simulink model "sampleModel20"  (R2021a)
settings: Solver=VariableStepAuto  StartTime=0.0  StopTime=10.0  RelTol=1e-3
undefined symbols (not defined in the file): DiscIntNeverNeededParam, magnitude, Newton, Raphson
libraries: simulink x274, pid_lib x17
(part 9 of 16)

== system sampleModel20/cfblk77/cfblk5/cfblk9/cfblk9 ==
  cfblk1 : Inport
  cfblk10 : Inport  Port=2
  cfblk3 : Math  Operator=mod  SaturateOnIntegerOverflow=on
  cfblk4 : Sum  Inputs=|++
  cfblk5 : Bias  Bias=[-186657263.890599]
  cfblk6 : Abs
  cfblk7 : Bias  Bias=[-144051976.581815]
  cfblk8 : Sum  Inputs=|++
  cfblk9 : simulink/Math Operations/MinMax Running Resettable  Function=min  vinit=0.0
  cfblk2 : Outport
  wires:
  cfblk10/1 -> cfblk6/1
  cfblk8/1 -> cfblk3/1
  cfblk9/1 -> cfblk5/1
  cfblk1/1 -> cfblk8/1
  cfblk5/1 -> cfblk2/1
  cfblk4/1 -> cfblk8/2
  cfblk6/1 -> cfblk7/1, cfblk4/2, cfblk3/2
  cfblk7/1 -> cfblk9/1, cfblk4/1
  cfblk3/1 -> cfblk9/2

== system sampleModel20/cfblk77/cfblk6/cfblk5/cfblk9 ==
  cfblk1 : Inport
  cfblk7 : Inport  Port=2
  cfblk8 : Inport  Port=3
  cfblk9 : Inport  Port=4
  cfblk13 : Delay  SampleTime=1
  cfblk14 : Delay  SampleTime=1
  cfblk3 : DiscreteTransferFcn  SampleTime=1
  cfblk4 : ComplexToRealImag
  cfblk5 : Gain  Gain=[186657996.322162]
  cfblk6 : Sum  Inputs=+
  cfblk2 : Outport
  cfblk10 : Outport  Port=2
  cfblk11 : Outport  Port=3
  cfblk12 : Outport  Port=4
  wires:
  cfblk3/1 -> cfblk5/1
  cfblk7/1 -> cfblk2/1
  cfblk8/1 -> cfblk11/1
  cfblk4/1 -> cfblk6/1
  cfblk9/1 -> cfblk10/1
  cfblk4/2 -> cfblk12/1
  cfblk5/1 -> cfblk13/1
  cfblk13/1 -> cfblk3/1
  cfblk6/1 -> cfblk14/1
  cfblk14/1 -> cfblk4/1

== system sampleModel20/cfblk77/cfblk6/cfblk6/cfblk6 ==
  cfblk1 : Inport
  cfblk4 : Inport  Port=2
  cfblk5 : Inport  Port=3
  cfblk6 : Inport  Port=4
  cfblk3 : Sin  TimeSource=Use external signal  SampleTime=0
  cfblk2 : Outport
  cfblk7 : Outport  Port=2
  wires:
  cfblk5/1 -> cfblk3/1
  cfblk1/1 -> cfblk2/1
  cfblk6/1 -> cfblk7/1

== system sampleModel20/cfblk77/cfblk6/cfblk6/cfblk7 ==
  cfblk1 : Inport
  cfblk10 : Inport  Port=2
  cfblk11 : Inport  Port=3
  cfblk12 : Inport  Port=4
  cfblk13 : Inport  Port=5
  cfblk14 : Inport  Port=6
  cfblk3 : ComplexToRealImag
  cfblk4 : Sqrt  Operator=rSqrt  AlgorithmType=Newton-Raphson  SaturateOnIntegerOverflow=on
  cfblk5 : PermuteDimensions
  cfblk6 : Reshape
  cfblk7 : Sum  Inputs=+
  cfblk8 : Product  Inputs=*
  cfblk9 : Sum  Inputs=|++
  cfblk2 : Outport
  cfblk15 : Outport  Port=2
  wires:
  cfblk13/1 -> cfblk15/1
  cfblk3/1 -> cfblk4/1
  cfblk10/1 -> cfblk8/1
  cfblk1/1 -> cfblk7/1
  cfblk9/1 -> cfblk5/1
  cfblk3/2 -> cfblk9/1
  cfblk5/1 -> cfblk6/1
  cfblk7/1 -> cfblk2/1
  cfblk12/1 -> cfblk3/1
  cfblk4/1 -> cfblk9/2

== system sampleModel20/cfblk77/cfblk6/cfblk6/cfblk8 ==
  cfblk1 : Inport
  cfblk12 : Inport  Port=2
  cfblk13 : Inport  Port=3
  cfblk14 : Inport  Port=4
  cfblk15 : Inport  Port=5
  cfblk16 : Inport  Port=6
  cfblk10 : Sum  Inputs=+-
  cfblk11 : Gain  Gain=[-598651231.399179]
  cfblk18 : Delay  SampleTime=1
  cfblk3 : Product  Inputs=**
  cfblk4 : Product  Inputs=**
  cfblk5 : Assignment  DiagnosticForDimensions=Warning  IndexOptions=Index vector (dialog)  Indices=1  OutputSizes=1
  cfblk6 : Assignment  DiagnosticForDimensions=Warning  IndexOptions=Index vector (dialog)  Indices=1  OutputSizes=1
  cfblk7 : Abs
  cfblk8 : Bias  Bias=[-168883268.146316]
  cfblk9 : Sum  Inputs=|++
  cfblk2 : Outport
  cfblk17 : Outport  Port=2
  wires:
  cfblk15/1 -> cfblk9/1
  cfblk14/1 -> cfblk3/1
  cfblk16/1 -> cfblk6/1, cfblk10/2
  cfblk5/1 -> cfblk11/1
  cfblk13/1 -> cfblk17/1
  cfblk4/1 -> cfblk6/2
  cfblk12/1 -> cfblk5/1
  cfblk11/1 -> cfblk2/1
  cfblk1/1 -> cfblk9/2
  cfblk10/1 -> cfblk4/2
  cfblk6/1 -> cfblk8/1
  cfblk9/1 -> cfblk7/1
  cfblk3/1 -> cfblk10/1
  cfblk7/1 -> cfblk3/2, cfblk5/2
  cfblk8/1 -> cfblk18/1
  cfblk18/1 -> cfblk4/1

== system sampleModel20/cfblk77/cfblk6/cfblk7/cfblk11 ==
  cfblk1 : Inport
  cfblk8 : Inport  Port=2
  cfblk9 : Inport  Port=3
  cfblk10 : Inport  Port=4
  cfblk11 : Inport  Port=5
  cfblk12 : Inport  Port=6
  cfblk3 : simulink/Math Operations/Slider Gain  gain=1  low=0  high=2
  cfblk4 : Sum  Inputs=|++
  cfblk5 : Sqrt  SaturateOnIntegerOverflow=on
  cfblk6 : ComplexToRealImag
  cfblk7 : Rounding
  cfblk2 : Outport
  cfblk13 : Outport  Port=2
  wires:
  cfblk6/1 -> cfblk7/1
  cfblk5/1 -> cfblk6/1
  cfblk8/1 -> cfblk2/1
  cfblk12/1 -> cfblk5/1
  cfblk10/1 -> cfblk4/1
  cfblk1/1 -> cfblk4/2
  cfblk11/1 -> cfblk3/1
  cfblk9/1 -> cfblk13/1

== system sampleModel20/cfblk77/cfblk6/cfblk7/cfblk12 ==
  cfblk1 : Inport
  cfblk7 : Inport  Port=2
  cfblk8 : Inport  Port=3
  cfblk3 : Reshape
  cfblk4 : Sum  Inputs=|++
  cfblk5 : Rounding
  cfblk6 : Sqrt  Operator=rSqrt  AlgorithmType=Newton-Raphson  SaturateOnIntegerOverflow=on
  cfblk9 : Delay  SampleTime=1
  cfblk2 : Outport
  wires:
  cfblk8/1 -> cfblk2/1
  cfblk5/1 -> cfblk4/1
  cfblk1/1 -> cfblk5/1
  cfblk7/1 -> cfblk3/1
  cfblk4/1 -> cfblk6/1
  cfblk6/1 -> cfblk9/1
  cfblk9/1 -> cfblk4/2

== system sampleModel20/cfblk77/cfblk6/cfblk8/cfblk8 ==
  cfblk1 : Inport
  cfblk5 : Inport  Port=2
  cfblk6 : Inport  Port=3
  cfblk7 : Inport  Port=4
  cfblk8 : Inport  Port=5
  cfblk9 : Inport  Port=6
  cfblk10 : Inport  Port=7
  cfblk3 : Product  Inputs=*
  cfblk4 : simulink/Math Operations/MinMax Running Resettable  Function=min  vinit=0.0
  cfblk2 : Outport
  cfblk11 : Outport  Port=2
  wires:
  cfblk4/1 -> cfblk3/1
  cfblk5/1 -> cfblk2/1
  cfblk10/1 -> cfblk4/1
  cfblk9/1 -> cfblk11/1
  cfblk1/1 -> cfblk4/2

== system sampleModel20/cfblk77/cfblk6/cfblk8/cfblk9 ==
  cfblk1 : Inport
  cfblk4 : Inport  Port=2
  cfblk5 : Inport  Port=3
  cfblk6 : Inport  Port=4
  cfblk3 : Bias  Bias=[-292302917.614101]
  cfblk2 : Outport
  cfblk7 : Outport  Port=2
  wires:
  cfblk4/1 -> cfblk2/1
  cfblk6/1 -> cfblk7/1
  cfblk5/1 -> cfblk3/1

== system sampleModel20/cfblk77/cfblk6/cfblk9/cfblk7 ==
  cfblk1 : Inport
  cfblk6 : Inport  Port=2
  cfblk7 : Inport  Port=3
  cfblk8 : Inport  Port=4
  cfblk9 : Inport  Port=5
  cfblk10 : Inport  Port=6
  cfblk11 : Inport  Port=7
  cfblk3 : MinMax  Function=max  Inputs=3
  cfblk4 : Product
  cfblk5 : Trigonometry
  cfblk2 : Outport
  cfblk12 : Outport  Port=2
  cfblk13 : Outport  Port=3
  cfblk14 : Outport  Port=4
  wires:
  cfblk1/1 -> cfblk5/1
  cfblk4/1 -> cfblk12/1
  cfblk5/1 -> cfblk4/1
  cfblk6/1 -> cfblk4/2
  cfblk10/1 -> cfblk3/1
  cfblk3/1 -> cfblk13/1
  cfblk7/1 -> cfblk2/1
  cfblk11/1 -> cfblk14/1
  cfblk9/1 -> cfblk3/2
  cfblk8/1 -> cfblk3/3

== system sampleModel20/cfblk77/cfblk6/cfblk9/cfblk8 ==
  cfblk1 : Inport
  cfblk5 : Inport  Port=2
  cfblk6 : Inport  Port=3
  cfblk3 : Squeeze
  cfblk4 : ComplexToMagnitudeAngle
  cfblk2 : Outport
  cfblk7 : Outport  Port=2
  wires:
  cfblk1/1 -> cfblk7/1
  cfblk4/1 -> cfblk2/1
  cfblk5/1 -> cfblk3/1
  cfblk3/1 -> cfblk4/1

== system sampleModel20/cfblk77/cfblk7/cfblk10/cfblk10 ==
  cfblk1 : Inport
  cfblk6 : Inport  Port=2
  cfblk7 : Inport  Port=3
  cfblk8 : Inport  Port=4
  cfblk9 : Inport  Port=5
  cfblk3 : simulink/Math Operations/MinMax Running Resettable  Function=min  vinit=0.0
  cfblk4 : ComplexToMagnitudeAngle
  cfblk5 : Gain  Gain=[652238342.291025]
  cfblk2 : Outport
  wires:
  cfblk4/1 -> cfblk5/1
  cfblk9/1 -> cfblk4/1
  cfblk4/2 -> cfblk2/1
  cfblk5/1 -> cfblk3/1
  cfblk7/1 -> cfblk3/2

== system sampleModel20/cfblk77/cfblk7/cfblk10/cfblk11 ==
  cfblk1 : Inport
  cfblk5 : Inport  Port=2
  cfblk6 : Inport  Port=3
  cfblk3 : Delay  ShowEnablePort=on  SampleTime=1
      settings: InputPortMap=u0,e6
  cfblk4 : UnaryMinus
  cfblk8 : Delay  SampleTime=1
  cfblk2 : Outport
  cfblk7 : Outport  Port=2
  wires:
  cfblk3/1 -> cfblk4/1
  cfblk5/1 -> cfblk7/1
  cfblk1/1 -> cfblk2/1
  cfblk6/1 -> cfblk3/1
  cfblk4/1 -> cfblk8/1
  cfblk8/1 -> cfblk3/2

== system sampleModel20/cfblk77/cfblk7/cfblk10/cfblk12 ==
  cfblk1 : Inport
  cfblk12 : Inport  Port=2
  cfblk13 : Inport  Port=3
  cfblk14 : Inport  Port=4
  cfblk10 : Polyval  Coefs=[ +2.081618890e-019, -1.441693666e-014, +4.719686976e-010, -8.536869453e-006, +1.621573104e-001, -8.087801117e+001 ]
  cfblk11 : Abs
  cfblk3 : pid_lib/PID Controller  Controller=PID  Form=Parallel  TimeDomain=Discrete-time  UseExternalTs=off  SampleTime=1  IntegratorMethod=Forward Euler  FilterMethod=Forward Euler  ControllerParametersSource=internal  P=1  I=1  D=0  UseFilter=on  N=100  TunerSelectOption=Transfer Function Based (PID Tuner App)  InitialConditionSource=internal  InitialConditionForIntegrator=0  InitialConditionForFilter=0  DifferentiatorICPrevScaledInput=0  ExternalReset=none  TrackingMode=off  Kt=1  LimitOutput=off  SatLimitsSource=internal  UpperSaturationLimit=inf  LowerSaturationLimit=-inf  LinearizeAsGain=off  AntiWindupMode=none  Kb=1  POutMin=[]  POutMax=[]  IOutMin=[]  IOutMax=[]  DOutMin=[]  DOutMax=[]  NOutMin=[]  NOutMax=[]  SumOutMin=[]  SumOutMax=[]  SaturationOutMin=[]  SaturationOutMax=[]  PParamMin=[]  PParamMax=[]  IParamMin=[]  IParamMax=[]  DParamMin=[]  DParamMax=[]  NParamMin=[]  NParamMax=[]  KbParamMin=[]  KbParamMax=[]  KtParamMin=[]  KtParamMax=[]  KbOutMin=[]  KbOutMax=[]  KtOutMin=[]  KtOutMax=[]  IntegratorOutMin=[]  IntegratorOutMax=[]  FilterOutMin=[]  FilterOutMax=[]  SumI1OutMin=[]  SumI1OutMax=[]  SumI2OutMin=[]  SumI2OutMax=[]  SumI3OutMin=[]  SumI3OutMax=[]  SumI4OutMin=[]  SumI4OutMax=[]  SumDOutMin=[]  SumDOutMax=[]  DifferentiatorOutMin=[]  DifferentiatorOutMax=[]  FilterDiffOutCoefMin=[]  FilterDiffOutCoefMax=[]  ReciprocalOutMin=[]  ReciprocalOutMax=[]  SumDenOutMin=[]  SumDenOutMax=[]  SumNumOutMin=[]  SumNumOutMax=[]  DivideOutMin=[]  DivideOutMax=[]  UdiffTsProdOutMin=[]  UdiffTsProdOutMax=[]  NTsProdOutMin=[]  NTsProdOutMax=[]  UintegralTsProdOutMin=[]  UintegralTsProdOutMax=[]  UngainTsProdOutMin=[]  UngainTsProdOutMax=[]  IntegratorContinuousStateAttributes=''  IntegratorStateMustResolveToSignalObject=off  IntegratorRTWStateStorageClass=Auto  FilterContinuousStateAttributes=''  FilterStateMustResolveToSignalObject=off  FilterRTWStateStorageClass=Auto  ParallelPVariant=InternalParameters  IdealPVariant=Disabled  IVariant=InternalParameters  DVariant=InternalParameters  IntegratorVariant=Discrete  SatVariant=Disabled  AWVariant=Passthrough  PCopyVariant=Disabled  TRVariant=Disabled  FdbkBlocksVariant=Forward  IdealPFdbkVariant=Disabled  SatFdbkVariant=Disabled  DerivativeFilterVariant=ForwardEulerFilter  NVariant=InternalParameters  NCopyVariant=Disabled  FilterICVariant=InternalICsFilter  IntegratorICVariant=InternalICs  ExternalResetVariant=Disabled  TRSumVariant=Passthrough  SumFdbkVariant=Disabled  SumVariant=Sum_PID  TsampFilterVariant=InternalTs  TsampNgainVariant=Passthrough  TsampIntegralVariant=Passthrough  ExternalSaturationOutDataTypeStr=Inherit: Same as second input
  cfblk4 : Product  Inputs=*
  cfblk5 : Squeeze
  cfblk6 : PermuteDimensions
  cfblk7 : Squeeze
  cfblk8 : Product  Inputs=*
  cfblk9 : ComplexToMagnitudeAngle
  cfblk2 : Outport
  cfblk15 : Outport  Port=2
  cfblk16 : Outport  Port=3
  cfblk17 : Outport  Port=4
  wires:
  cfblk3/1 -> cfblk9/1
  cfblk4/1 -> cfblk8/1
  cfblk5/1 -> cfblk11/1
  cfblk11/1 -> cfblk3/1
  cfblk1/1 -> cfblk6/1
  cfblk14/1 -> cfblk15/1
  cfblk8/1 -> cfblk7/1
  cfblk7/1 -> cfblk16/1
  cfblk6/1 -> cfblk2/1
  cfblk12/1 -> cfblk5/1
  cfblk13/1 -> cfblk10/1
  cfblk9/1 -> cfblk17/1
  cfblk9/2 -> cfblk4/1

== system sampleModel20/cfblk77/cfblk7/cfblk10/cfblk13 ==
  cfblk1 : Inport
  cfblk9 : Inport  Port=2
  cfblk10 : Inport  Port=3
  cfblk11 : Inport  Port=4
  cfblk12 : Inport  Port=5
  cfblk13 : Inport  Port=6
  cfblk14 : Inport  Port=7
  cfblk3 : simulink/Discrete/Difference  ICPrevInput=0.0  OutMin=[]  OutMax=[]  OutDataTypeStr=Inherit: Inherit via back propagation  OutDataType=fixdt(1, 16)  OutScaling=2^-10  DoSatur=off
  cfblk4 : Sqrt  Operator=rSqrt  AlgorithmType=Newton-Raphson  SaturateOnIntegerOverflow=on
  cfblk5 : Sum  Inputs=|++
  cfblk6 : Trigonometry
  cfblk7 : ComplexToMagnitudeAngle
  cfblk8 : UnaryMinus
  cfblk2 : Outport
  cfblk15 : Outport  Port=2
  cfblk16 : Outport  Port=3
  cfblk17 : Outport  Port=4
  wires:
  cfblk13/1 -> cfblk17/1
  cfblk1/1 -> cfblk8/1
  cfblk10/1 -> cfblk5/1
  cfblk8/1 -> cfblk3/1
  cfblk12/1 -> cfblk15/1
  cfblk9/1 -> cfblk4/1
  cfblk11/1 -> cfblk16/1
  cfblk14/1 -> cfblk7/1
  cfblk4/1 -> cfblk6/1
  cfblk7/1 -> cfblk5/2
  cfblk6/1 -> cfblk2/1

== system sampleModel20/cfblk77/cfblk7/cfblk10/cfblk9 ==
  cfblk1 : Inport
  cfblk8 : Inport  Port=2
  cfblk9 : Inport  Port=3
  cfblk10 : Inport  Port=4
  cfblk11 : Inport  Port=5
  cfblk12 : Inport  Port=6
  cfblk13 : Inport  Port=7
  cfblk14 : Delay  SampleTime=1
  cfblk3 : Reshape
  cfblk4 : Sin  TimeSource=Use external signal  SampleTime=0
  cfblk5 : Abs
  cfblk6 : Bias  Bias=[-31221541.110679]
  cfblk7 : Product
  cfblk2 : Outport
  wires:
  cfblk1/1 -> cfblk2/1
  cfblk11/1 -> cfblk6/1
  cfblk13/1 -> cfblk7/1
  cfblk12/1 -> cfblk4/1
  cfblk3/1 -> cfblk7/2
  cfblk10/1 -> cfblk5/1
  cfblk7/1 -> cfblk14/1
  cfblk14/1 -> cfblk3/1

== system sampleModel20/cfblk77/cfblk7/cfblk8/cfblk7 ==
  cfblk1 : Inport
  cfblk7 : Inport  Port=2
  cfblk8 : Inport  Port=3
  cfblk9 : Inport  Port=4
  cfblk10 : Inport  Port=5
  cfblk11 : Inport  Port=6
  cfblk12 : Inport  Port=7
  cfblk13 : Inport  Port=8
  cfblk3 : DiscreteFir  SampleTime=1
  cfblk4 : Gain  Gain=[-495455232.000155]
  cfblk5 : Squeeze
  cfblk6 : ComplexToMagnitudeAngle
  cfblk2 : Outport
  cfblk14 : Outport  Port=2
  wires:
  cfblk11/1 -> cfblk5/1
  cfblk8/1 -> cfblk6/1
  cfblk1/1 -> cfblk3/1
  cfblk9/1 -> cfblk4/1
  cfblk5/1 -> cfblk2/1
  cfblk7/1 -> cfblk14/1

== system sampleModel20/cfblk77/cfblk7/cfblk8/cfblk8 ==
  cfblk1 : Inport
  cfblk5 : Inport  Port=2
  cfblk6 : Inport  Port=3
  cfblk7 : Inport  Port=4
  cfblk8 : Inport  Port=5
  cfblk3 : Math  Operator=mod  SaturateOnIntegerOverflow=on
  cfblk4 : Rounding
  cfblk2 : Outport
  cfblk9 : Outport  Port=2
  wires:
  cfblk4/1 -> cfblk3/1
  cfblk7/1 -> cfblk3/2
  cfblk1/1 -> cfblk9/1
  cfblk8/1 -> cfblk4/1
  cfblk6/1 -> cfblk2/1

== system sampleModel20/cfblk77/cfblk7/cfblk8/cfblk9 ==
  cfblk1 : Inport
  cfblk7 : Inport  Port=2
  cfblk8 : Inport  Port=3
  cfblk3 : simulink/Math Operations/Slider Gain  gain=1  low=0  high=2
  cfblk4 : Polyval  Coefs=[ +2.081618890e-019, -1.441693666e-014, +4.719686976e-010, -8.536869453e-006, +1.621573104e-001, -8.087801117e+001 ]
  cfblk5 : DotProduct  InputSameDT=on  OutDataTypeStr=Inherit: Inherit via internal rule
  cfblk6 : ComplexToRealImag
  cfblk2 : Outport
  cfblk9 : Outport  Port=2
  wires:
  cfblk7/1 -> cfblk3/1
  cfblk1/1 -> cfblk6/1
  cfblk6/1 -> cfblk2/1
  cfblk6/2 -> cfblk4/1
  cfblk3/1 -> cfblk5/1
  cfblk8/1 -> cfblk9/1
  cfblk4/1 -> cfblk5/2

== system sampleModel20/cfblk77/cfblk7/cfblk9/cfblk18 ==
  cfblk1 : Inport
  cfblk6 : Inport  Port=2
  cfblk7 : Inport  Port=3
  Action Port : ActionPort  ActionPortLabel=if(u1 >= 0)
  cfblk3 : ComplexToMagnitudeAngle
  cfblk4 : PermuteDimensions
  cfblk5 : Polyval  Coefs=[ +2.081618890e-019, -1.441693666e-014, +4.719686976e-010, -8.536869453e-006, +1.621573104e-001, -8.087801117e+001 ]
  cfblk2 : Outport
  wires:
  cfblk6/1 -> cfblk5/1
  cfblk5/1 -> cfblk4/1
  cfblk3/1 -> cfblk2/1
  cfblk7/1 -> cfblk3/1

== system sampleModel20/cfblk77/cfblk7/cfblk9/cfblk19 ==
  cfblk1 : Inport
  cfblk6 : Inport  Port=2
  cfblk7 : Inport  Port=3
  Action Port : ActionPort  ActionPortLabel=else
  cfblk3 : Product  Inputs=*
  cfblk4 : Sin  TimeSource=Use external signal  SampleTime=0
  cfblk5 : MinMax  Inputs=3
  cfblk2 : Outport
  wires:
  cfblk1/1 -> cfblk3/1
  cfblk6/1 -> cfblk4/1
  cfblk3/1 -> cfblk2/1
  cfblk4/1 -> cfblk5/1
  cfblk7/1 -> cfblk5/2, cfblk5/3

== system sampleModel20/cfblk77/cfblk7/cfblk9/cfblk8 ==
  cfblk1 : Inport
  cfblk10 : Inport  Port=2
  cfblk11 : Inport  Port=3
  cfblk12 : Inport  Port=4
  cfblk13 : Inport  Port=5
  cfblk14 : Inport  Port=6
  cfblk3 : Trigonometry
  cfblk4 : Polyval  Coefs=[ +2.081618890e-019, -1.441693666e-014, +4.719686976e-010, -8.536869453e-006, +1.621573104e-001, -8.087801117e+001 ]
  cfblk5 : Assignment  DiagnosticForDimensions=Warning  IndexOptions=Index vector (dialog)  Indices=1  OutputSizes=1
  cfblk6 : Trigonometry
  cfblk7 : Product
  cfblk8 : Signum
  cfblk9 : Reshape
  cfblk2 : Outport
  cfblk15 : Outport  Port=2
  wires:
  cfblk4/1 -> cfblk6/1
  cfblk5/1 -> cfblk15/1
  cfblk6/1 -> cfblk7/1
  cfblk14/1 -> cfblk4/1
  cfblk11/1 -> cfblk3/1
  cfblk1/1 -> cfblk9/1
  cfblk8/1 -> cfblk2/1
  cfblk3/1 -> cfblk7/2
  cfblk9/1 -> cfblk8/1
  cfblk10/1 -> cfblk5/1
  cfblk7/1 -> cfblk5/2

== system sampleModel20/cfblk77/cfblk7/cfblk9/cfblk9 ==
  cfblk1 : Inport
  cfblk11 : Inport  Port=2
  cfblk12 : Inport  Port=3
  cfblk13 : Inport  Port=4
  cfblk14 : Inport  Port=5
  cfblk10 : simulink/Math Operations/MinMax Running Resettable  Function=min  vinit=0.0
  cfblk3 : Reshape
  cfblk4 : Squeeze
  cfblk5 : Sqrt  SaturateOnIntegerOverflow=on
  cfblk6 : Sum  Inputs=+
  cfblk7 : Assignment  DiagnosticForDimensions=Warning  IndexOptions=Index vector (dialog)  Indices=1  OutputSizes=1
  cfblk8 : Abs
  cfblk9 : simulink/Math Operations/MinMax Running Resettable  Function=min  vinit=0.0
  cfblk2 : Outport
  cfblk15 : Outport  Port=2
  cfblk16 : Outport  Port=3
  cfblk17 : Outport  Port=4
  wires:
  cfblk3/1 -> cfblk16/1
  cfblk11/1 -> cfblk9/1
  cfblk12/1 -> cfblk7/1
  cfblk8/1 -> cfblk2/1
  cfblk1/1 -> cfblk4/1
  cfblk13/1 -> cfblk5/1
  cfblk7/1 -> cfblk8/1
  cfblk5/1 -> cfblk10/1
  cfblk4/1 -> cfblk9/2, cfblk7/2
  cfblk14/1 -> cfblk15/1
  cfblk6/1 -> cfblk17/1
  cfblk9/1 -> cfblk10/2
  cfblk10/1 -> cfblk6/1, cfblk3/1

== system sampleModel20/cfblk77/cfblk8/cfblk10/cfblk7 ==
  cfblk1 : Inport
  cfblk6 : Inport  Port=2
  cfblk7 : Inport  Port=3
  cfblk8 : Inport  Port=4
  cfblk9 : Inport  Port=5
  cfblk10 : Inport  Port=6
  cfblk11 : Inport  Port=7
  cfblk12 : Inport  Port=8
  cfblk15 : Delay  SampleTime=1
  cfblk3 : Sum  Inputs=+-
  cfblk4 : Product  Inputs=*
  cfblk5 : DotProduct  InputSameDT=on  OutDataTypeStr=Inherit: Inherit via internal rule
  cfblk2 : Outport
  cfblk13 : Outport  Port=2
  cfblk14 : Outport  Port=3
  wires:
  cfblk5/1 -> cfblk4/1
  cfblk6/1 -> cfblk14/1
  cfblk12/1 -> cfblk3/1
  cfblk7/1 -> cfblk13/1
  cfblk1/1 -> cfblk5/1
  cfblk8/1 -> cfblk2/1
  cfblk11/1 -> cfblk3/2
  cfblk4/1 -> cfblk15/1
  cfblk15/1 -> cfblk5/2

== system sampleModel20/cfblk77/cfblk8/cfblk10/cfblk8 ==
  cfblk1 : Inport
  cfblk9 : Inport  Port=2
  cfblk10 : Inport  Port=3
  cfblk11 : Inport  Port=4
  cfblk14 : Delay  SampleTime=1
  cfblk15 : Delay  SampleTime=1
  cfblk3 : Product
  cfblk4 : ComplexToMagnitudeAngle
  cfblk5 : Squeeze
  cfblk6 : ComplexToMagnitudeAngle
  cfblk7 : simulink/Math Operations/Slider Gain  gain=1  low=0  high=2
  cfblk8 : ComplexToMagnitudeAngle
  cfblk2 : Outport
  cfblk12 : Outport  Port=2
  cfblk13 : Outport  Port=3
  wires:
  cfblk5/1 -> cfblk2/1
  cfblk3/1 -> cfblk8/1
  cfblk6/1 -> cfblk3/2
  cfblk6/2 -> cfblk7/1
  cfblk11/1 -> cfblk5/1
  cfblk4/1 -> cfblk13/1
  cfblk1/1 -> cfblk12/1
  cfblk9/1 -> cfblk4/1
  cfblk8/1 -> cfblk14/1
  cfblk14/1 -> cfblk3/1
  cfblk7/1 -> cfblk15/1
  cfblk15/1 -> cfblk6/1

== system sampleModel20/cfblk77/cfblk8/cfblk5/cfblk5 ==
  cfblk1 : Inport
  cfblk8 : Inport  Port=2
  cfblk9 : Inport  Port=3
  cfblk10 : Inport  Port=4
  cfblk11 : Inport  Port=5
  cfblk3 : Product  Inputs=**
  cfblk4 : DotProduct  InputSameDT=on  OutDataTypeStr=Inherit: Inherit via internal rule
  cfblk5 : Gain  Gain=[-153420040.522857]
  cfblk6 : Sum  Inputs=|++
  cfblk7 : ComplexToMagnitudeAngle
  cfblk2 : Outport
  wires:
  cfblk11/1 -> cfblk5/1
  cfblk1/1 -> cfblk3/1
  cfblk6/1 -> cfblk7/1
  cfblk7/1 -> cfblk3/2
  cfblk10/1 -> cfblk6/1
  cfblk8/1 -> cfblk2/1
  cfblk9/1 -> cfblk6/2
  cfblk5/1 -> cfblk4/1
  cfblk7/2 -> cfblk4/2

== system sampleModel20/cfblk77/cfblk8/cfblk5/cfblk6 ==
  cfblk1 : Inport
  cfblk5 : Inport  Port=2
  cfblk6 : Inport  Port=3
  cfblk7 : Inport  Port=4
  cfblk3 : Product  Inputs=*
  cfblk4 : simulink/Math Operations/MinMax Running Resettable  Function=min  vinit=0.0
  cfblk2 : Outport
  cfblk8 : Outport  Port=2
  wires:
  cfblk6/1 -> cfblk2/1
  cfblk3/1 -> cfblk8/1
  cfblk7/1 -> cfblk3/1
  cfblk1/1 -> cfblk4/1
  cfblk5/1 -> cfblk4/2

== system sampleModel20/cfblk77/cfblk8/cfblk5/cfblk7 ==
  cfblk1 : Inport
  cfblk8 : Inport  Port=2
  cfblk9 : Inport  Port=3
  cfblk12 : Delay  SampleTime=1
  cfblk3 : ComplexToRealImag
  cfblk4 : Squeeze
  cfblk5 : Sqrt  SaturateOnIntegerOverflow=on
  cfblk6 : MinMax  Inputs=3
  cfblk7 : simulink/Math Operations/Slider Gain  gain=1  low=0  high=2
  cfblk2 : Outport
  cfblk10 : Outport  Port=2
  cfblk11 : Outport  Port=3
  wires:
  cfblk3/1 -> cfblk7/1
  cfblk8/1 -> cfblk11/1
  cfblk9/1 -> cfblk4/1
  cfblk7/1 -> cfblk10/1
  cfblk4/1 -> cfblk3/1
  cfblk1/1 -> cfblk6/2, cfblk6/3
  cfblk3/2 -> cfblk2/1
  cfblk6/1 -> cfblk5/1
  cfblk5/1 -> cfblk12/1
  cfblk12/1 -> cfblk6/1

== system sampleModel20/cfblk77/cfblk8/cfblk5/cfblk8 ==
  cfblk1 : Inport
  cfblk8 : Inport  Port=2
  cfblk9 : Inport  Port=3
  cfblk10 : Inport  Port=4
  cfblk11 : Inport  Port=5
  cfblk12 : Inport  Port=6
  cfblk14 : Delay  SampleTime=1
  cfblk3 : Product  Inputs=**
  cfblk4 : Sum  Inputs=+-
  cfblk5 : simulink/Math Operations/MinMax Running Resettable  Function=min  vinit=0.0
  cfblk6 : Sum  Inputs=--
  cfblk7 : UnaryMinus
  cfblk2 : Outport
  cfblk13 : Outport  Port=2
  wires:
  cfblk10/1 -> cfblk5/1
  cfblk7/1 -> cfblk2/1
  cfblk6/1 -> cfblk4/1
  cfblk8/1 -> cfblk13/1
  cfblk1/1 -> cfblk7/1
  cfblk4/1 -> cfblk5/2
  cfblk11/1 -> cfblk3/2
  cfblk9/1 -> cfblk4/2
  cfblk3/1 -> cfblk6/1
  cfblk12/1 -> cfblk6/2
  cfblk5/1 -> cfblk14/1
  cfblk14/1 -> cfblk3/1

== system sampleModel20/cfblk77/cfblk8/cfblk6/cfblk10 ==
  cfblk1 : Inport
  cfblk5 : Inport  Port=2
  cfblk6 : Inport  Port=3
  cfblk3 : Trigonometry
  cfblk4 : simulink/Math Operations/MinMax Running Resettable  Function=min  vinit=0.0
  cfblk2 : Outport
  cfblk7 : Outport  Port=2
  wires:
  cfblk6/1 -> cfblk4/1
  cfblk4/1 -> cfblk3/1
  cfblk3/1 -> cfblk7/1
  cfblk5/1 -> cfblk2/1
  cfblk1/1 -> cfblk4/2

== system sampleModel20/cfblk77/cfblk8/cfblk6/cfblk8 ==
  cfblk1 : Inport
  cfblk8 : Inport  Port=2
  cfblk9 : Inport  Port=3
  cfblk10 : Inport  Port=4
  cfblk11 : Inport  Port=5
  cfblk3 : Abs
  cfblk4 : ComplexToMagnitudeAngle
  cfblk5 : Product  Inputs=*
  cfblk6 : Sin  TimeSource=Use external signal  SampleTime=0
  cfblk7 : Reshape
  cfblk2 : Outport
  wires:
  cfblk1/1 -> cfblk5/1
  cfblk9/1 -> cfblk6/1
  cfblk7/1 -> cfblk4/1
  cfblk11/1 -> cfblk7/1
  cfblk8/1 -> cfblk2/1
  cfblk10/1 -> cfblk3/1

== system sampleModel20/cfblk77/cfblk8/cfblk6/cfblk9 ==
  cfblk1 : Inport
  cfblk13 : Inport  Port=2
  cfblk14 : Inport  Port=3
  cfblk15 : Inport  Port=4
  cfblk10 : Polyval  Coefs=[ +2.081618890e-019, -1.441693666e-014, +4.719686976e-010, -8.536869453e-006, +1.621573104e-001, -8.087801117e+001 ]
  cfblk11 : Math  Operator=transpose  SaturateOnIntegerOverflow=on
  cfblk12 : Sum  Inputs=+-
  cfblk3 : ComplexToRealImag
  cfblk4 : Sqrt  Operator=rSqrt  AlgorithmType=Newton-Raphson  SaturateOnIntegerOverflow=on
  cfblk5 : Sqrt  SaturateOnIntegerOverflow=on
  cfblk6 : simulink/Math Operations/Slider Gain  gain=1  low=0  high=2
  cfblk7 : DotProduct  InputSameDT=on  OutDataTypeStr=Inherit: Inherit via internal rule
  cfblk8 : Squeeze
  cfblk9 : Rounding
  cfblk2 : Outport
  cfblk16 : Outport  Port=2
  wires:
  cfblk3/1 -> cfblk5/1
  cfblk5/1 -> cfblk7/1
  cfblk3/2 -> cfblk6/1
  cfblk4/1 -> cfblk3/1
  cfblk1/1 -> cfblk16/1
  cfblk10/1 -> cfblk7/2
  cfblk14/1 -> cfblk8/1
  cfblk7/1 -> cfblk12/1
  cfblk15/1 -> cfblk4/1
  cfblk13/1 -> cfblk12/2
  cfblk6/1 -> cfblk11/1
  cfblk8/1 -> cfblk10/1
  cfblk12/1 -> cfblk2/1
  cfblk11/1 -> cfblk9/1

== system sampleModel20/cfblk77/cfblk8/cfblk7/cfblk10 ==
  cfblk1 : Inport
  cfblk9 : Inport  Port=2
  cfblk10 : Inport  Port=3
  cfblk11 : Inport  Port=4
  cfblk12 : Inport  Port=5
  cfblk13 : Inport  Port=6
  cfblk14 : Inport  Port=7
  cfblk15 : Inport  Port=8
  cfblk3 : PermuteDimensions
  cfblk4 : DotProduct  InputSameDT=on  OutDataTypeStr=Inherit: Inherit via internal rule
  cfblk5 : Math  SaturateOnIntegerOverflow=on
  cfblk6 : Bias  Bias=[941663766.223596]
  cfblk7 : Polyval  Coefs=[ +2.081618890e-019, -1.441693666e-014, +4.719686976e-010, -8.536869453e-006, +1.621573104e-001, -8.087801117e+001 ]
  cfblk8 : DotProduct  InputSameDT=on  OutDataTypeStr=Inherit: Inherit via internal rule
  cfblk2 : Outport
  cfblk16 : Outport  Port=2
  wires:
  cfblk7/1 -> cfblk4/1
  cfblk15/1 -> cfblk3/1
  cfblk10/1 -> cfblk16/1
  cfblk6/1 -> cfblk2/1
  cfblk11/1 -> cfblk4/2
  cfblk9/1 -> cfblk8/1
  cfblk1/1 -> cfblk7/1
  cfblk13/1 -> cfblk8/2
  cfblk12/1 -> cfblk5/1
  cfblk3/1 -> cfblk6/1

== system sampleModel20/cfblk77/cfblk8/cfblk7/cfblk8 ==
  cfblk1 : Inport
  cfblk8 : Inport  Port=2
  cfblk9 : Inport  Port=3
  cfblk10 : Inport  Port=4
  cfblk11 : Inport  Port=5
  cfblk12 : Inport  Port=6
  cfblk13 : Inport  Port=7
  cfblk14 : Inport  Port=8
  cfblk3 : Sqrt  SaturateOnIntegerOverflow=on
  cfblk4 : simulink/Math Operations/MinMax Running Resettable  Function=min  vinit=0.0
  cfblk5 : Signum
  cfblk6 : Signum
  cfblk7 : simulink/Math Operations/Slider Gain  gain=1  low=0  high=2
  cfblk2 : Outport
  cfblk15 : Outport  Port=2
  wires:
  cfblk13/1 -> cfblk15/1
  cfblk9/1 -> cfblk7/1
  cfblk14/1 -> cfblk4/1
  cfblk7/1 -> cfblk4/2
  cfblk4/1 -> cfblk5/1
  cfblk10/1 -> cfblk3/1
  cfblk12/1 -> cfblk6/1
  cfblk5/1 -> cfblk2/1

== system sampleModel20/cfblk77/cfblk8/cfblk7/cfblk9 ==
  cfblk1 : Inport
  cfblk10 : Inport  Port=2
  cfblk11 : Inport  Port=3
  cfblk12 : Inport  Port=4
  cfblk13 : Inport  Port=5
  cfblk14 : Inport  Port=6
  cfblk16 : Delay  SampleTime=1
  cfblk3 : Reshape
  cfblk4 : UnaryMinus
  cfblk5 : Reshape
  cfblk6 : Sqrt  Operator=rSqrt  AlgorithmType=Newton-Raphson  SaturateOnIntegerOverflow=on
  cfblk7 : Sum  Inputs=+-
  cfblk8 : Assignment  DiagnosticForDimensions=Warning  IndexOptions=Index vector (dialog)  Indices=1  OutputSizes=1
  cfblk9 : Rounding
  cfblk2 : Outport
  cfblk15 : Outport  Port=2
  wires:
  cfblk12/1 -> cfblk7/1
  cfblk11/1 -> cfblk4/1
  cfblk9/1 -> cfblk3/1
  cfblk3/1 -> cfblk2/1
  cfblk10/1 -> cfblk9/1
  cfblk5/1 -> cfblk6/1
  cfblk1/1 -> cfblk15/1
  cfblk6/1 -> cfblk8/1
  cfblk7/1 -> cfblk8/2
  cfblk13/1 -> cfblk7/2
  cfblk8/1 -> cfblk16/1
  cfblk16/1 -> cfblk5/1

== system sampleModel20/cfblk77/cfblk8/cfblk8/cfblk10 ==
  cfblk1 : Inport
  cfblk9 : Inport  Port=2
  cfblk10 : Inport  Port=3
  cfblk11 : Inport  Port=4
  cfblk12 : Inport  Port=5
  cfblk13 : Inport  Port=6
  cfblk15 : Delay  SampleTime=1
  cfblk16 : Delay  SampleTime=1
  cfblk3 : UnaryMinus
  cfblk4 : Math  Operator=log  SaturateOnIntegerOverflow=on
  cfblk5 : Sqrt  Operator=rSqrt  AlgorithmType=Newton-Raphson  SaturateOnIntegerOverflow=on
  cfblk6 : Product
  cfblk7 : UnaryMinus
  cfblk8 : Polyval  Coefs=[ +2.081618890e-019, -1.441693666e-014, +4.719686976e-010, -8.536869453e-006, +1.621573104e-001, -8.087801117e+001 ]
  cfblk2 : Outport
  cfblk14 : Outport  Port=2
  wires:
  cfblk1/1 -> cfblk6/1
  cfblk5/1 -> cfblk8/1
  cfblk7/1 -> cfblk3/1
  cfblk13/1 -> cfblk14/1
  cfblk6/1 -> cfblk7/1
  cfblk12/1 -> cfblk4/1
  cfblk11/1 -> cfblk2/1
  cfblk3/1 -> cfblk15/1
  cfblk15/1 -> cfblk6/2
  cfblk8/1 -> cfblk16/1
  cfblk16/1 -> cfblk5/1

== system sampleModel20/cfblk77/cfblk8/cfblk8/cfblk7 ==
  cfblk1 : Inport
  cfblk6 : Inport  Port=2
  cfblk7 : Inport  Port=3
  cfblk3 : Sum  Inputs=+-
  cfblk4 : Sum  Inputs=+
  cfblk5 : Reshape
  cfblk2 : Outport
  cfblk8 : Outport  Port=2
  cfblk9 : Outport  Port=3
  wires:
  cfblk7/1 -> cfblk3/1
  cfblk3/1 -> cfblk4/1, cfblk8/1
  cfblk1/1 -> cfblk5/1
  cfblk6/1 -> cfblk3/2
  cfblk5/1 -> cfblk2/1
  cfblk4/1 -> cfblk9/1

== system sampleModel20/cfblk77/cfblk8/cfblk8/cfblk8 ==
  cfblk1 : Inport
  cfblk9 : Inport  Port=2
  cfblk10 : Delay  SampleTime=1
  cfblk3 : UnaryMinus
  cfblk4 : PermuteDimensions
  cfblk5 : Sum  Inputs=|++
  cfblk6 : Reshape
  cfblk7 : Signum
  cfblk8 : Trigonometry
  cfblk2 : Outport
  wires:
  cfblk3/1 -> cfblk6/1
  cfblk4/1 -> cfblk8/1
  cfblk5/1 -> cfblk2/1
  cfblk1/1 -> cfblk5/1
  cfblk6/1 -> cfblk4/1
  cfblk7/1 -> cfblk5/2
  cfblk9/1 -> cfblk7/1
  cfblk8/1 -> cfblk10/1
  cfblk10/1 -> cfblk3/1

== system sampleModel20/cfblk77/cfblk8/cfblk8/cfblk9 ==
  cfblk1 : Inport
  cfblk4 : Inport  Port=2
  cfblk5 : Inport  Port=3
  cfblk6 : Inport  Port=4
  cfblk3 : Polyval  Coefs=[ +2.081618890e-019, -1.441693666e-014, +4.719686976e-010, -8.536869453e-006, +1.621573104e-001, -8.087801117e+001 ]
  cfblk2 : Outport
  cfblk7 : Outport  Port=2
  wires:
  cfblk1/1 -> cfblk7/1
  cfblk5/1 -> cfblk2/1
  cfblk6/1 -> cfblk3/1

== system sampleModel20/cfblk77/cfblk8/cfblk9/cfblk5 ==
  cfblk1 : Inport
  cfblk10 : Inport  Port=2
  cfblk11 : Inport  Port=3
  cfblk12 : Inport  Port=4
  cfblk13 : Inport  Port=5
  cfblk14 : Inport  Port=6
  cfblk15 : Inport  Port=7
  cfblk3 : Sqrt  Operator=rSqrt  AlgorithmType=Newton-Raphson  SaturateOnIntegerOverflow=on
  cfblk4 : Sin  TimeSource=Use external signal  SampleTime=0
  cfblk5 : simulink/Math Operations/Slider Gain  gain=1  low=0  high=2
  cfblk6 : Product
  cfblk7 : Signum
  cfblk8 : UnaryMinus
  cfblk9 : DotProduct  InputSameDT=on  OutDataTypeStr=Inherit: Inherit via internal rule
  cfblk2 : Outport
  cfblk16 : Outport  Port=2
  wires:
  cfblk14/1 -> cfblk4/1
  cfblk7/1 -> cfblk2/1
  cfblk10/1 -> cfblk7/1
  cfblk15/1 -> cfblk9/1
  cfblk13/1 -> cfblk6/1
  cfblk8/1 -> cfblk5/1
  cfblk1/1 -> cfblk6/2
  cfblk12/1 -> cfblk9/2
  cfblk3/1 -> cfblk8/1
  cfblk4/1 -> cfblk3/1
  cfblk5/1 -> cfblk16/1

== system sampleModel20/cfblk77/cfblk8/cfblk9/cfblk6 ==
  cfblk1 : Inport
  cfblk11 : Inport  Port=2
  cfblk12 : Inport  Port=3
  cfblk13 : Inport  Port=4
  cfblk10 : Signum
  cfblk15 : Delay  SampleTime=1
  cfblk3 : DiscreteStateSpace
  cfblk4 : Sum  Inputs=|++
  cfblk5 : ComplexToMagnitudeAngle
  cfblk6 : ComplexToRealImag
  cfblk7 : Sum  Inputs=+-
  cfblk8 : Signum
  cfblk9 : Gain  Gain=[496330480.796783]
  cfblk2 : Outport
  cfblk14 : Outport  Port=2
  wires:
  cfblk4/1 -> cfblk7/1
  cfblk13/1 -> cfblk8/1
  cfblk3/1 -> cfblk5/1
  cfblk8/1 -> cfblk7/2
  cfblk5/1 -> cfblk6/1
  cfblk9/1 -> cfblk4/2
  cfblk1/1 -> cfblk14/1
  cfblk12/1 -> cfblk10/1
  cfblk11/1 -> cfblk3/1
  cfblk5/2 -> cfblk9/1
  cfblk6/1 -> cfblk2/1
  cfblk7/1 -> cfblk15/1
  cfblk15/1 -> cfblk4/1

== system sampleModel20/cfblk77/cfblk9/cfblk5/cfblk6 ==
  cfblk1 : Inport
  cfblk5 : Inport  Port=2
  cfblk6 : Inport  Port=3
  cfblk7 : Inport  Port=4
  cfblk3 : Squeeze
  cfblk4 : Product  Inputs=**
  cfblk2 : Outport
  wires:
  cfblk7/1 -> cfblk3/1
  cfblk1/1 -> cfblk2/1
  cfblk6/1 -> cfblk4/1
  cfblk3/1 -> cfblk4/2

== system sampleModel20/cfblk77/cfblk9/cfblk6/cfblk10 ==
  cfblk1 : Inport
  cfblk7 : Inport  Port=2
  cfblk8 : Inport  Port=3
  cfblk9 : Inport  Port=4
  cfblk10 : Inport  Port=5
  cfblk11 : Inport  Port=6
  cfblk12 : Inport  Port=7
  cfblk13 : Inport  Port=8
  cfblk14 : Inport  Port=9
  cfblk15 : Inport  Port=10
  cfblk3 : Sum  Inputs=|++
  cfblk4 : PermuteDimensions
  cfblk5 : DotProduct  InputSameDT=on  OutDataTypeStr=Inherit: Inherit via internal rule
  cfblk6 : ComplexToRealImag
  cfblk2 : Outport
  cfblk16 : Outport  Port=2
  wires:
  cfblk15/1 -> cfblk2/1
  cfblk9/1 -> cfblk4/1
  cfblk3/1 -> cfblk6/1
  cfblk14/1 -> cfblk5/1
  cfblk10/1 -> cfblk16/1
  cfblk12/1 -> cfblk5/2
  cfblk11/1 -> cfblk3/1
  cfblk7/1 -> cfblk3/2

== system sampleModel20/cfblk77/cfblk9/cfblk6/cfblk11 ==
  cfblk1 : Inport
  cfblk7 : Inport  Port=2
  cfblk8 : Inport  Port=3
  cfblk9 : Inport  Port=4
  cfblk10 : Inport  Port=5
  cfblk11 : Inport  Port=6
  cfblk12 : Delay  SampleTime=1
  cfblk3 : DotProduct  InputSameDT=on  OutDataTypeStr=Inherit: Inherit via internal rule
  cfblk4 : simulink/Math Operations/MinMax Running Resettable  Function=min  vinit=0.0
  cfblk5 : ComplexToRealImag
  cfblk6 : Product
  cfblk2 : Outport
  wires:
  cfblk11/1 -> cfblk4/1
  cfblk9/1 -> cfblk3/1
  cfblk1/1 -> cfblk6/2
  cfblk7/1 -> cfblk2/1
  cfblk5/1 -> cfblk4/2
  cfblk8/1 -> cfblk5/1
  cfblk6/1 -> cfblk3/2
  cfblk3/1 -> cfblk12/1
  cfblk12/1 -> cfblk6/1

== system sampleModel20/cfblk77/cfblk9/cfblk6/cfblk9 ==
  cfblk1 : Inport
  cfblk6 : Inport  Port=2
  cfblk7 : Inport  Port=3
  cfblk8 : Inport  Port=4
  cfblk3 : Sqrt  Operator=rSqrt  AlgorithmType=Newton-Raphson  SaturateOnIntegerOverflow=on
  cfblk4 : DotProduct  InputSameDT=on  OutDataTypeStr=Inherit: Inherit via internal rule
  cfblk5 : Sum  Inputs=+
  cfblk2 : Outport
  cfblk9 : Outport  Port=2
  wires:
  cfblk3/1 -> cfblk9/1
  cfblk6/1 -> cfblk3/1
  cfblk4/1 -> cfblk2/1
  cfblk1/1 -> cfblk5/1
  cfblk5/1 -> cfblk4/1
  cfblk8/1 -> cfblk4/2

== system sampleModel20/cfblk78/cfblk10/cfblk7/cfblk6 ==
  cfblk1 : Inport
  cfblk9 : Inport  Port=2
  cfblk10 : Inport  Port=3
  cfblk11 : Inport  Port=4
  cfblk12 : Inport  Port=5
  cfblk13 : Inport  Port=6
  cfblk3 : Product
  cfblk4 : simulink/Math Operations/MinMax Running Resettable  Function=min  vinit=0.0
  cfblk5 : Product  Inputs=*
  cfblk6 : Math  Operator=log  SaturateOnIntegerOverflow=on
  cfblk7 : ComplexToMagnitudeAngle
  cfblk8 : Sum  Inputs=+-
  cfblk2 : Outport
  wires:
  cfblk12/1 -> cfblk3/1
  cfblk1/1 -> cfblk6/1
  cfblk6/1 -> cfblk7/1
  cfblk3/1 -> cfblk4/1
  cfblk13/1 -> cfblk4/2
  cfblk4/1 -> cfblk5/1
  cfblk11/1 -> cfblk3/2
  cfblk9/1 -> cfblk2/1
  cfblk10/1 -> cfblk8/1
  cfblk5/1 -> cfblk8/2

== system sampleModel20/cfblk78/cfblk10/cfblk7/cfblk7 ==
  cfblk1 : Inport
  cfblk12 : Inport  Port=2
  cfblk13 : Inport  Port=3
  cfblk14 : Inport  Port=4
  cfblk15 : Inport  Port=5
  cfblk16 : Inport  Port=6
  cfblk10 : Bias  Bias=[704712383.954292]
  cfblk11 : Assignment  DiagnosticForDimensions=Warning  IndexOptions=Index vector (dialog)  Indices=1  OutputSizes=1
  cfblk18 : Delay  SampleTime=1
  cfblk3 : Product  Inputs=*
  cfblk4 : Sin  TimeSource=Use external signal  SampleTime=0
  cfblk5 : Math  Operator=pow  SaturateOnIntegerOverflow=on
  cfblk6 : Squeeze
  cfblk7 : ComplexToRealImag
  cfblk8 : DotProduct  InputSameDT=on  OutDataTypeStr=Inherit: Inherit via internal rule
  cfblk9 : ComplexToMagnitudeAngle
  cfblk2 : Outport
  cfblk17 : Outport  Port=2
  wires:
  cfblk11/1 -> cfblk3/1
  cfblk6/1 -> cfblk8/1
  cfblk15/1 -> cfblk8/2
  cfblk13/1 -> cfblk6/1
  cfblk3/1 -> cfblk4/1
  cfblk14/1 -> cfblk9/1
  cfblk8/1 -> cfblk17/1
  cfblk12/1 -> cfblk10/1
  cfblk5/1 -> cfblk7/1
  cfblk9/1 -> cfblk11/1
  cfblk10/1 -> cfblk2/1
  cfblk7/2 -> cfblk11/2
  cfblk16/1 -> cfblk5/2
  cfblk7/1 -> cfblk18/1
  cfblk18/1 -> cfblk5/1

== system sampleModel20/cfblk78/cfblk10/cfblk7/cfblk8 ==
  cfblk1 : Inport
  cfblk12 : Inport  Port=2
  cfblk13 : Inport  Port=3
  cfblk14 : Inport  Port=4
  cfblk15 : Inport  Port=5
  cfblk10 : Product  Inputs=*
  cfblk11 : Bias  Bias=[3689681.794733]
  cfblk17 : Delay  SampleTime=1
  cfblk18 : Delay  SampleTime=1
  cfblk3 : simulink/Discrete/Tapped Delay  vinit=0.0  samptime=-1  NumDelays=1  DelayOrder=Oldest  includeCurrent=off
  cfblk4 : ComplexToMagnitudeAngle
  cfblk5 : ComplexToMagnitudeAngle
  cfblk6 : Bias  Bias=[-516115041.402766]
  cfblk7 : Product  Inputs=**
  cfblk8 : Sqrt  SaturateOnIntegerOverflow=on
  cfblk9 : Squeeze
  cfblk2 : Outport
  cfblk16 : Outport  Port=2
  wires:
  cfblk12/1 -> cfblk16/1
  cfblk10/1 -> cfblk8/1
  cfblk3/1 -> cfblk9/1
  cfblk4/1 -> cfblk11/1
  cfblk5/1 -> cfblk7/1
  cfblk6/1 -> cfblk5/1
  cfblk9/1 -> cfblk10/1
  cfblk1/1 -> cfblk6/1
  cfblk15/1 -> cfblk7/2
  cfblk5/2 -> cfblk2/1
  cfblk8/1 -> cfblk17/1
  cfblk17/1 -> cfblk3/1
  cfblk11/1 -> cfblk18/1
  cfblk18/1 -> cfblk4/1

== system sampleModel20/cfblk78/cfblk7/cfblk6/cfblk5 ==
  cfblk1 : Inport
  cfblk9 : Inport  Port=2
  cfblk10 : Inport  Port=3
  cfblk11 : Inport  Port=4
  cfblk12 : Inport  Port=5
  cfblk13 : Inport  Port=6
  cfblk14 : Inport  Port=7
  cfblk15 : Inport  Port=8
  cfblk3 : DiscreteFilter  SampleTime=1
  cfblk4 : Product  Inputs=**
  cfblk5 : Math  Operator=magnitude^2  SaturateOnIntegerOverflow=on
  cfblk6 : Rounding
  cfblk7 : simulink/Math Operations/Slider Gain  gain=1  low=0  high=2
  cfblk8 : Product  Inputs=**
  cfblk2 : Outport
  wires:
  cfblk7/1 -> cfblk5/1
  cfblk11/1 -> cfblk3/1
  cfblk9/1 -> cfblk7/1
  cfblk3/1 -> cfblk8/1
  cfblk8/1 -> cfblk6/1
  cfblk10/1 -> cfblk8/2
  cfblk1/1 -> cfblk2/1
  cfblk6/1 -> cfblk4/1
  cfblk14/1 -> cfblk4/2

== system sampleModel20/cfblk78/cfblk7/cfblk6/cfblk6 ==
  cfblk1 : Inport
  cfblk7 : Inport  Port=2
  cfblk10 : Delay  SampleTime=1
  cfblk3 : Product  Inputs=**
  cfblk4 : Sqrt  SaturateOnIntegerOverflow=on
  cfblk5 : Sum  Inputs=|++
  cfblk6 : Trigonometry
  cfblk2 : Outport
  cfblk8 : Outport  Port=2
  cfblk9 : Outport  Port=3
  wires:
  cfblk4/1 -> cfblk5/1
  cfblk7/1 -> cfblk8/1, cfblk3/2
  cfblk1/1 -> cfblk2/1, cfblk5/2
  cfblk5/1 -> cfblk9/1
  cfblk3/1 -> cfblk4/1, cfblk6/1
  cfblk6/1 -> cfblk10/1
  cfblk10/1 -> cfblk3/1

== system sampleModel20/cfblk78/cfblk7/cfblk6/cfblk7 ==
  cfblk1 : Inport
  cfblk6 : Inport  Port=2
  cfblk7 : Inport  Port=3
  cfblk8 : Inport  Port=4
  cfblk9 : Inport  Port=5
  cfblk10 : Inport  Port=6
  cfblk11 : Inport  Port=7
  cfblk12 : Inport  Port=8
  cfblk13 : Inport  Port=9
  cfblk14 : Inport  Port=10
  cfblk3 : Abs
  cfblk4 : Sum  Inputs=+-
  cfblk5 : simulink/Math Operations/MinMax Running Resettable  Function=min  vinit=0.0
  cfblk2 : Outport
  wires:
  cfblk12/1 -> cfblk3/1
  cfblk11/1 -> cfblk2/1
  cfblk3/1 -> cfblk5/1
  cfblk10/1 -> cfblk4/1
  cfblk7/1 -> cfblk4/2
  cfblk14/1 -> cfblk5/2

== system sampleModel20/cfblk78/cfblk7/cfblk6/cfblk8 ==
  cfblk1 : Inport
  cfblk4 : Inport  Port=2
  cfblk5 : Inport  Port=3
  cfblk6 : Inport  Port=4
  cfblk7 : Inport  Port=5
  cfblk8 : Inport  Port=6
  cfblk9 : Inport  Port=7
  cfblk10 : Inport  Port=8
  cfblk3 : Abs
  cfblk2 : Outport
  cfblk11 : Outport  Port=2
  wires:
  cfblk4/1 -> cfblk2/1
  cfblk6/1 -> cfblk11/1
  cfblk5/1 -> cfblk3/1

== system sampleModel20/cfblk78/cfblk7/cfblk7/cfblk6 ==
  cfblk1 : Inport
  cfblk5 : Inport  Port=2
  cfblk6 : Inport  Port=3
  cfblk7 : Inport  Port=4
  cfblk3 : Sqrt  SaturateOnIntegerOverflow=on
  cfblk4 : Product
  cfblk2 : Outport
  cfblk8 : Outport  Port=2
  cfblk9 : Outport  Port=3
  wires:
  cfblk1/1 -> cfblk8/1
  cfblk7/1 -> cfblk9/1
  cfblk5/1 -> cfblk3/1
  cfblk6/1 -> cfblk4/1
  cfblk3/1 -> cfblk4/2
  cfblk4/1 -> cfblk2/1

== system sampleModel20/cfblk78/cfblk7/cfblk7/cfblk7 ==
  cfblk1 : Inport
  cfblk6 : Inport  Port=2
  cfblk7 : Inport  Port=3
  cfblk8 : Inport  Port=4
  cfblk9 : Inport  Port=5
  cfblk10 : Inport  Port=6
  cfblk3 : Sum
  cfblk4 : Sin  TimeSource=Use external signal  SampleTime=0
  cfblk5 : Signum
  cfblk2 : Outport
  wires:
  cfblk6/1 -> cfblk5/1
  cfblk3/1 -> cfblk2/1
  cfblk4/1 -> cfblk3/1
  cfblk9/1 -> cfblk4/1
  cfblk8/1 -> cfblk3/2

== system sampleModel20/cfblk78/cfblk8/cfblk5/cfblk11 ==
  cfblk1 : Inport
  cfblk10 : Inport  Port=2
  cfblk11 : Inport  Port=3
  cfblk13 : Delay  SampleTime=1
  cfblk3 : DiscreteStateSpace
  cfblk4 : Sqrt  SaturateOnIntegerOverflow=on
  cfblk5 : Bias  Bias=[-517799713.728035]
  cfblk6 : PermuteDimensions
  cfblk7 : Sum  Inputs=|++
  cfblk8 : Polyval  Coefs=[ +2.081618890e-019, -1.441693666e-014, +4.719686976e-010, -8.536869453e-006, +1.621573104e-001, -8.087801117e+001 ]
  cfblk9 : Bias  Bias=[261002689.464966]
  cfblk2 : Outport
  cfblk12 : Outport  Port=2
  wires:
  cfblk10/1 -> cfblk4/1
  cfblk7/1 -> cfblk5/1
  cfblk6/1 -> cfblk9/1
  cfblk1/1 -> cfblk8/1
  cfblk4/1 -> cfblk6/1
  cfblk8/1 -> cfblk7/2
  cfblk9/1 -> cfblk12/1
  cfblk11/1 -> cfblk3/1
  cfblk3/1 -> cfblk2/1
  cfblk5/1 -> cfblk13/1
  cfblk13/1 -> cfblk7/1

== system sampleModel20/cfblk78/cfblk8/cfblk5/cfblk12 ==
  cfblk1 : Inport
  cfblk12 : Inport  Port=2
  cfblk13 : Inport  Port=3
  cfblk14 : Inport  Port=4
  cfblk10 : Product  Inputs=*
  cfblk11 : MinMax  Inputs=3
  cfblk{3,18..20} (4 alike) : Delay  SampleTime=1
  cfblk4 : Sin  TimeSource=Use external signal  SampleTime=0
  cfblk5 : DotProduct  InputSameDT=on  OutDataTypeStr=Inherit: Inherit via internal rule
  cfblk6 : Sin  TimeSource=Use external signal  SampleTime=0
  cfblk7 : Sum  Inputs=+
  cfblk8 : Abs
  cfblk9 : Abs
  cfblk2 : Outport
  cfblk15 : Outport  Port=2
  cfblk16 : Outport  Port=3
  cfblk17 : Outport  Port=4
  wires:
  cfblk6/1 -> cfblk9/1, cfblk11/2
  cfblk1/1 -> cfblk17/1
  cfblk10/1 -> cfblk4/1
  cfblk4/1 -> cfblk18/1, cfblk19/1
  cfblk8/1 -> cfblk15/1
  cfblk14/1 -> cfblk7/1
  cfblk11/1 -> cfblk10/1
  cfblk3/1 -> cfblk11/1
  cfblk7/1 -> cfblk16/1, cfblk5/2
  cfblk13/1 -> cfblk2/1
  cfblk12/1 -> cfblk5/1
  cfblk5/1 -> cfblk8/1
  cfblk18/1 -> cfblk3/1
  cfblk19/1 -> cfblk11/3
  cfblk9/1 -> cfblk20/1
  cfblk20/1 -> cfblk6/1

== system sampleModel20/cfblk78/cfblk8/cfblk5/cfblk13 ==
  cfblk1 : Inport
  cfblk5 : Inport  Port=2
  cfblk6 : Inport  Port=3
  cfblk3 : Sin  TimeSource=Use external signal  SampleTime=0
  cfblk4 : Sqrt  Operator=rSqrt  AlgorithmType=Newton-Raphson  SaturateOnIntegerOverflow=on
  cfblk2 : Outport
  cfblk7 : Outport  Port=2
  wires:
  cfblk1/1 -> cfblk4/1
  cfblk3/1 -> cfblk2/1
  cfblk5/1 -> cfblk7/1
  cfblk4/1 -> cfblk3/1

== system sampleModel20/cfblk78/cfblk8/cfblk6/cfblk6 ==
  cfblk1 : Inport
  cfblk5 : Inport  Port=2
  cfblk6 : Inport  Port=3
  cfblk7 : Inport  Port=4
  cfblk8 : Inport  Port=5
  cfblk9 : Inport  Port=6
  cfblk10 : Inport  Port=7
  cfblk11 : Inport  Port=8
  cfblk3 : Sum  Inputs=+-
  cfblk4 : DotProduct  InputSameDT=on  OutDataTypeStr=Inherit: Inherit via internal rule
  cfblk2 : Outport
  cfblk12 : Outport  Port=2
  cfblk13 : Outport  Port=3
  wires:
  cfblk9/1 -> cfblk3/1
  cfblk11/1 -> cfblk3/2
  cfblk1/1 -> cfblk13/1
  cfblk5/1 -> cfblk2/1
  cfblk7/1 -> cfblk4/1
  cfblk3/1 -> cfblk12/1
  cfblk8/1 -> cfblk4/2

== system sampleModel20/cfblk78/cfblk8/cfblk6/cfblk7 ==
  cfblk1 : Inport
  cfblk6 : Inport  Port=2
  cfblk7 : Inport  Port=3
  cfblk8 : Inport  Port=4
  cfblk9 : Inport  Port=5
  cfblk10 : Inport  Port=6
  cfblk11 : Inport  Port=7
  cfblk3 : Product  Inputs=**
  cfblk4 : Reshape
  cfblk5 : Product
  cfblk2 : Outport
  cfblk12 : Outport  Port=2
  wires:
  cfblk10/1 -> cfblk12/1
  cfblk8/1 -> cfblk5/1
  cfblk5/1 -> cfblk2/1
  cfblk7/1 -> cfblk3/1
  cfblk9/1 -> cfblk5/2
  cfblk1/1 -> cfblk3/2
  cfblk3/1 -> cfblk4/1

== system sampleModel20/cfblk78/cfblk9/cfblk10/cfblk8 ==
  cfblk1 : Inport
  cfblk9 : Inport  Port=2
  cfblk10 : Inport  Port=3
  cfblk11 : Inport  Port=4
  cfblk12 : Inport  Port=5
  cfblk13 : Inport  Port=6
  cfblk14 : Inport  Port=7
  cfblk3 : simulink/Math Operations/Slider Gain  gain=1  low=0  high=2
  cfblk4 : Bias  Bias=[-489855605.608294]
  cfblk5 : Product  Inputs=*
  cfblk6 : simulink/Math Operations/Slider Gain  gain=1  low=0  high=2
  cfblk7 : simulink/Math Operations/MinMax Running Resettable  Function=min  vinit=0.0
  cfblk8 : Trigonometry
  cfblk2 : Outport
  wires:
  cfblk12/1 -> cfblk7/1
  cfblk4/1 -> cfblk3/1
  cfblk1/1 -> cfblk4/1
  cfblk7/1 -> cfblk6/1
  cfblk11/1 -> cfblk8/1
  cfblk5/1 -> cfblk7/2
  cfblk14/1 -> cfblk5/1
  cfblk3/1 -> cfblk2/1

== system sampleModel20/cfblk78/cfblk9/cfblk10/cfblk9 ==
  cfblk1 : Inport
  cfblk11 : Inport  Port=2
  cfblk12 : Inport  Port=3
  cfblk13 : Inport  Port=4
  cfblk14 : Inport  Port=5
  cfblk10 : MinMax  Function=max  Inputs=2
  cfblk16 : Delay  SampleTime=1
  cfblk3 : Sum  Inputs=+
  cfblk4 : Polyval  Coefs=[ +2.081618890e-019, -1.441693666e-014, +4.719686976e-010, -8.536869453e-006, +1.621573104e-001, -8.087801117e+001 ]
  cfblk5 : Sqrt  SaturateOnIntegerOverflow=on
  cfblk6 : Abs
  cfblk7 : Reshape
  cfblk8 : Assignment  DiagnosticForDimensions=Warning  IndexOptions=Index vector (dialog)  Indices=1  OutputSizes=1
  cfblk9 : DotProduct  InputSameDT=on  OutDataTypeStr=Inherit: Inherit via internal rule
  cfblk2 : Outport
  cfblk15 : Outport  Port=2
  wires:
  cfblk14/1 -> cfblk6/1
  cfblk3/1 -> cfblk7/1
  cfblk11/1 -> cfblk2/1
  cfblk12/1 -> cfblk3/1
  cfblk9/1 -> cfblk4/1
  cfblk13/1 -> cfblk9/1
  cfblk7/1 -> cfblk5/1
  cfblk6/1 -> cfblk8/1
  cfblk4/1 -> cfblk10/2
  cfblk1/1 -> cfblk9/2
  cfblk5/1 -> cfblk15/1
  cfblk10/1 -> cfblk8/2
  cfblk8/1 -> cfblk16/1
  cfblk16/1 -> cfblk10/1

== system sampleModel20/cfblk78/cfblk9/cfblk11/cfblk5 ==
  cfblk1 : Inport
  cfblk10 : Inport  Port=2
  cfblk11 : Inport  Port=3
  cfblk12 : Inport  Port=4
  cfblk13 : Inport  Port=5
  cfblk14 : Inport  Port=6
  cfblk15 : Inport  Port=7
  cfblk16 : Inport  Port=8
  cfblk17 : Inport  Port=9
  cfblk3 : Abs
  cfblk4 : Sum  Inputs=+
  cfblk5 : Product
  cfblk6 : Product  Inputs=*
  cfblk7 : MinMax
  cfblk8 : MinMax  Inputs=3
  cfblk9 : Rounding
  cfblk2 : Outport
  wires:
  cfblk4/1 -> cfblk5/1
  cfblk12/1 -> cfblk8/1
  cfblk13/1 -> cfblk6/1
  cfblk9/1 -> cfblk2/1
  cfblk6/1 -> cfblk4/1
  cfblk1/1 -> cfblk7/1
  cfblk10/1 -> cfblk8/2
  cfblk7/1 -> cfblk3/1
  cfblk11/1 -> cfblk9/1
  cfblk15/1 -> cfblk8/3
  cfblk17/1 -> cfblk5/2

== system sampleModel20/cfblk78/cfblk9/cfblk11/cfblk6 ==
  cfblk1 : Inport
  cfblk5 : Inport  Port=2
  cfblk6 : Inport  Port=3
  cfblk3 : Bias  Bias=[371264225.337391]
  cfblk4 : Signum
  cfblk2 : Outport
  cfblk7 : Outport  Port=2
  wires:
  cfblk4/1 -> cfblk3/1
  cfblk6/1 -> cfblk4/1
  cfblk1/1 -> cfblk7/1
  cfblk5/1 -> cfblk2/1

== system sampleModel20/cfblk78/cfblk9/cfblk12/cfblk4 ==
  cfblk1 : Inport
  cfblk8 : Inport  Port=2
  cfblk9 : Inport  Port=3
  cfblk10 : Inport  Port=4
  cfblk11 : Inport  Port=5
  cfblk12 : Inport  Port=6
  cfblk13 : Inport  Port=7
  cfblk3 : PermuteDimensions
  cfblk4 : Polyval  Coefs=[ +2.081618890e-019, -1.441693666e-014, +4.719686976e-010, -8.536869453e-006, +1.621573104e-001, -8.087801117e+001 ]
  cfblk5 : Sum  Inputs=+-
  cfblk6 : Abs
  cfblk7 : Bias  Bias=[465831517.574610]
  cfblk2 : Outport
  cfblk14 : Outport  Port=2
  cfblk15 : Outport  Port=3
  wires:
  cfblk4/1 -> cfblk2/1
  cfblk7/1 -> cfblk6/1
  cfblk13/1 -> cfblk3/1
  cfblk9/1 -> cfblk15/1
  cfblk1/1 -> cfblk14/1
  cfblk11/1 -> cfblk4/1
  cfblk12/1 -> cfblk7/1
  cfblk3/1 -> cfblk5/1
  cfblk6/1 -> cfblk5/2

== system sampleModel20/cfblk78/cfblk9/cfblk12/cfblk5 ==
  cfblk1 : Inport
  cfblk4 : Inport  Port=2
  cfblk5 : Inport  Port=3
  cfblk6 : Inport  Port=4
  cfblk7 : Inport  Port=5
  cfblk3 : Product  Inputs=**
  cfblk2 : Outport
  cfblk8 : Outport  Port=2
  wires:
  cfblk7/1 -> cfblk8/1
  cfblk6/1 -> cfblk2/1
  cfblk5/1 -> cfblk3/1
  cfblk4/1 -> cfblk3/2

== system sampleModel20/cfblk78/cfblk9/cfblk12/cfblk6 ==
  cfblk1 : Inport
  cfblk6 : Inport  Port=2
  cfblk3 : Assignment  DiagnosticForDimensions=Warning  IndexOptions=Index vector (dialog)  Indices=1  OutputSizes=1
  cfblk4 : Sqrt  SaturateOnIntegerOverflow=on
  cfblk5 : Sqrt  Operator=rSqrt  AlgorithmType=Newton-Raphson  SaturateOnIntegerOverflow=on
  cfblk2 : Outport
  cfblk7 : Outport  Port=2
  wires:
  cfblk1/1 -> cfblk5/1, cfblk2/1
  cfblk3/1 -> cfblk7/1
  cfblk4/1 -> cfblk3/1
  cfblk5/1 -> cfblk3/2
  cfblk6/1 -> cfblk4/1

== system sampleModel20/cfblk78/cfblk9/cfblk12/cfblk7 ==
  cfblk1 : Inport
  cfblk9 : Inport  Port=2
  cfblk13 : Delay  SampleTime=1
  cfblk3 : Sqrt  Operator=rSqrt  AlgorithmType=Newton-Raphson  SaturateOnIntegerOverflow=on
  cfblk4 : Abs
  cfblk5 : Abs
  cfblk6 : Product
  cfblk7 : DotProduct  InputSameDT=on  OutDataTypeStr=Inherit: Inherit via internal rule
  cfblk8 : Product  Inputs=**
  cfblk2 : Outport
  cfblk10 : Outport  Port=2
  cfblk11 : Outport  Port=3
  cfblk12 : Outport  Port=4
  wires:
  cfblk4/1 -> cfblk8/1, cfblk7/1
  cfblk3/1 -> cfblk11/1, cfblk7/2
  cfblk6/1 -> cfblk2/1
  cfblk1/1 -> cfblk3/1
  cfblk9/1 -> cfblk5/1, cfblk6/2, cfblk12/1
  cfblk8/1 -> cfblk6/1, cfblk13/1
  cfblk5/1 -> cfblk8/2
  cfblk7/1 -> cfblk10/1
  cfblk13/1 -> cfblk4/1

== system sampleModel20/cfblk79/cfblk9/cfblk7/cfblk10 ==
  cfblk1 : Inport
  cfblk11 : Inport  Port=2
  cfblk12 : Inport  Port=3
  cfblk13 : Inport  Port=4
  cfblk14 : Inport  Port=5
  cfblk15 : Inport  Port=6
  cfblk16 : Inport  Port=7
  cfblk10 : UnaryMinus
  cfblk3 : MinMax  Function=max  Inputs=3
  cfblk4 : UnaryMinus
  cfblk5 : Sqrt  SaturateOnIntegerOverflow=on
  cfblk6 : Abs
  cfblk7 : Assignment  DiagnosticForDimensions=Warning  IndexOptions=Index vector (dialog)  Indices=1  OutputSizes=1
  cfblk8 : Product  Inputs=*
  cfblk9 : Math  Operator=rem  SaturateOnIntegerOverflow=on
  cfblk2 : Outport
  cfblk17 : Outport  Port=2
  wires:
  cfblk7/1 -> cfblk9/1
  cfblk11/1 -> cfblk3/1
  cfblk9/1 -> cfblk4/1
  cfblk8/1 -> cfblk7/1
  cfblk13/1 -> cfblk9/2
  cfblk12/1 -> cfblk3/2
  cfblk3/1 -> cfblk2/1
  cfblk4/1 -> cfblk10/1
  cfblk6/1 -> cfblk7/2
  cfblk10/1 -> cfblk3/3
  cfblk5/1 -> cfblk17/1
  cfblk15/1 -> cfblk8/1
  cfblk16/1 -> cfblk5/1
  cfblk14/1 -> cfblk6/1

== system sampleModel20/cfblk79/cfblk9/cfblk7/cfblk6 ==
  cfblk1 : Inport
  cfblk5 : Inport  Port=2
  cfblk6 : Inport  Port=3
  cfblk7 : Inport  Port=4
  cfblk8 : Inport  Port=5
  cfblk9 : Inport  Port=6
  cfblk10 : Inport  Port=7
  cfblk3 : MinMax  Inputs=3
  cfblk4 : Sqrt  SaturateOnIntegerOverflow=on
  cfblk2 : Outport
  cfblk11 : Outport  Port=2
  wires:
  cfblk8/1 -> cfblk3/1
  cfblk10/1 -> cfblk2/1
  cfblk3/1 -> cfblk11/1
  cfblk4/1 -> cfblk3/2
  cfblk5/1 -> cfblk4/1
  cfblk7/1 -> cfblk3/3

== system sampleModel20/cfblk79/cfblk9/cfblk7/cfblk7 ==
  cfblk1 : Inport
  cfblk4 : Inport  Port=2
  cfblk5 : Inport  Port=3
  cfblk6 : Inport  Port=4
  cfblk7 : Inport  Port=5
  cfblk8 : Inport  Port=6
  cfblk3 : DotProduct  InputSameDT=on  OutDataTypeStr=Inherit: Inherit via internal rule
  cfblk2 : Outport
  cfblk9 : Outport  Port=2
  cfblk10 : Outport  Port=3
  wires:
  cfblk4/1 -> cfblk2/1
  cfblk3/1 -> cfblk10/1
  cfblk8/1 -> cfblk3/1
  cfblk1/1 -> cfblk9/1
  cfblk5/1 -> cfblk3/2
